simulink model "DD202220405_homework"  (R2021a)
settings: Solver=VariableStepAuto  StartTime=0.0  StopTime=20  RelTol=1e-3
settings Model: Creator=jaewan  LastModifiedBy=jaewan

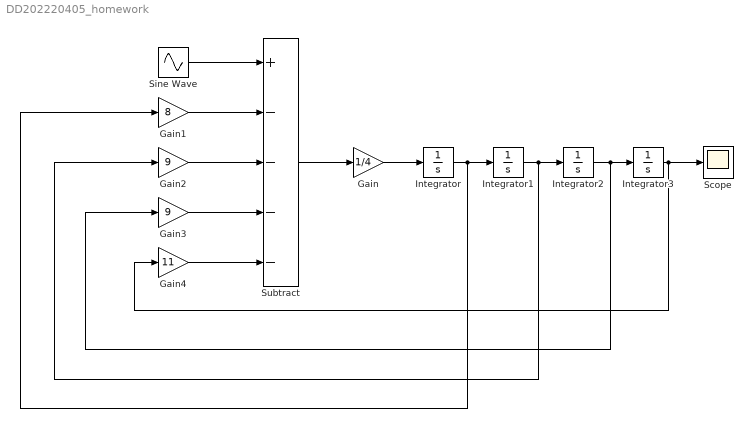
== system DD202220405_homework ==
  Gain : Gain  Gain=1/4
  Gain1 : Gain  Gain=8
  Gain2 : Gain  Gain=9
  Gain3 : Gain  Gain=9
  Gain4 : Gain  Gain=11
  Integrator{,1..3} (4 alike) : Integrator
  Scope : Scope
  Sine Wave : Sin  Amplitude=12  Frequency=5  SampleTime=0
  Subtract : Sum  Inputs=+----
  wires:
  Sine Wave/1 -> Subtract/1
  Gain1/1 -> Subtract/2
  Gain2/1 -> Subtract/3
  Gain/1 -> Integrator/1
  Subtract/1 -> Gain/1
  Integrator/1 -> Gain1/1, Integrator1/1
  Integrator1/1 -> Gain2/1, Integrator2/1
  Integrator2/1 -> Gain3/1, Integrator3/1
  Integrator3/1 -> Gain4/1, Scope/1
  Gain4/1 -> Subtract/5
  Gain3/1 -> Subtract/4
